simulink model "Integration_1_1"  (R2024b)
settings: Solver=VariableStepAuto  StartTime=0.0  StopTime=4  RelTol=1e-3
undefined symbols (not defined in the file): Ion, Lithium, Ts_Control
libraries: ee_lib x30, nesl_utility x24, spsSeriesRLCBranchLib x22, simulink x21, slpidlib x18, spsParallelRLCBranchLib x18, spsCurrentVoltageSimscapeInterfaceLib x18, powerlib_extras x18, spsThreePhaseVIMeasurementLib x7, spsGroundLib x7, spsThreePhaseSeriesRLCBranchLib x7, spsBoostConverterLib x6
(part 2 of 5)

== system Integration_1_1/Subsystem20 ==
  Series RLC Branch1 : spsSeriesRLCBranchLib/Series RLC Branch  LConnTagsString=__new0  RConnTagsString=__new0  BranchType=C  Resistance=10  Inductance=1e-3  SetiL0=off  InitialCurrent=0  Capacitance=1.316e-6  Setx0=off  InitialVoltage=0  Measurements=None
  Series RLC Branch2 : spsSeriesRLCBranchLib/Series RLC Branch  LConnTagsString=__new0  RConnTagsString=__new0  BranchType=C  Resistance=10  Inductance=1e-3  SetiL0=off  InitialCurrent=0  Capacitance=1.316e-6  Setx0=off  InitialVoltage=0  Measurements=None
  Series RLC Branch3 : spsSeriesRLCBranchLib/Series RLC Branch  LConnTagsString=__new0  RConnTagsString=__new0  BranchType=C  Resistance=10  Inductance=1e-3  SetiL0=off  InitialCurrent=0  Capacitance=1.316e-6  Setx0=off  InitialVoltage=0  Measurements=None
  Three-Phase Series RLC Branch1 : spsThreePhaseSeriesRLCBranchLib/Three-Phase Series RLC Branch  LConnTagsString=A|B|C  RConnTagsString=A|B|C  BranchType=L  Resistance=1  Inductance=3*2.309e-3  Capacitance=1e-6  Measurements=None
  A : PMIOPort  Side=Left
  B : PMIOPort  Port=2  Side=Left
  C : PMIOPort  Port=3  Side=Left
  a : PMIOPort  Port=4  Side=Right
  b : PMIOPort  Port=5  Side=Right
  c : PMIOPort  Port=6  Side=Right
  connections:
  Series RLC Branch2/LConn1 -- Series RLC Branch1/RConn1 -- c/RConn1 -- Three-Phase Series RLC Branch1/RConn3
  Three-Phase Series RLC Branch1/LConn3 -- C/RConn1
  Three-Phase Series RLC Branch1/LConn2 -- B/RConn1
  Three-Phase Series RLC Branch1/LConn1 -- A/RConn1
  Series RLC Branch2/RConn1 -- a/RConn1 -- Three-Phase Series RLC Branch1/RConn1 -- Series RLC Branch3/LConn1
  Series RLC Branch3/RConn1 -- b/RConn1 -- Three-Phase Series RLC Branch1/RConn2 -- Series RLC Branch1/LConn1

== system Integration_1_1/Subsystem3 ==
  Current-Voltage Simscape Interface : spsCurrentVoltageSimscapeInterfaceLib/Current-Voltage Simscape Interface  DFT=off  FMode=Low pass filter (continuous)  T=1e-4  Ts=50e-6  i0=0  v0=0  Sd=Specialized Power Systems side  Measurements=off
  Current-Voltage Simscape Interface1 : spsCurrentVoltageSimscapeInterfaceLib/Current-Voltage Simscape Interface  DFT=off  FMode=Low pass filter (continuous)  T=1e-4  Ts=50e-6  i0=0  v0=0  Sd=Specialized Power Systems side  Measurements=off
  Current-Voltage Simscape Interface2 : spsCurrentVoltageSimscapeInterfaceLib/Current-Voltage Simscape Interface  DFT=off  FMode=Low pass filter (continuous)  T=1e-4  Ts=50e-6  i0=0  v0=0  Sd=Specialized Power Systems side  Measurements=off
  Demux2 : Demux  Outputs=2
  Dynamic Load (Three-Phase) : ee_lib/Passive/Dynamic Load (Three-Phase)  port_option=ee.enum.threePhasePort.composite  FRated=50 Hz  Vline_rms_min=400 V  tau=0.01 s  Vline_rms_ini=400 V  Vang_ini=0 deg  gmin=0 S  fault_action=simscape.enum.assert.action.none  t_fault=1 s
      settings: InternalSimscapePortConfiguration="{\"Bottom\":[],\"Left\":[{\"id\":\"N\",\"label\":\"~\",\"type\":\"foundation.electrical.three_phase\"}],\"Right\":[],\"Top\":[{\"id\":\"P\",\"label\":\"P\",\"type\":\"input\"},{\"id\":\"Q\",\"label\":\"Q\",\"type\":\"input\"}]}"
  From Workspace5 : FromWorkspace  VariableName=load_data_32  SampleTime=0.01
  Ground3 : spsGroundLib/Ground  LConnTagsString=a
  Grounded Neutral (Three-Phase) : ee_lib/Connectors & References/Grounded Neutral (Three-Phase)
  PS-Simulink Converter : nesl_utility/PS-Simulink Converter  PhysicalDomain=network_engine_domain  SubClassName=ps_output  LeftPortType=input  RightPortType=output  PseudoPeriodic=off  Frequencies=[]  VectorFormat=inherit  Unit=inherit  AffineConversion=off
  Phase Splitter : ee_lib/Connectors & References/Phase Splitter
  Phase Splitter1 : ee_lib/Connectors & References/Phase Splitter
  Power Sensor (Three-Phase) : ee_lib/Sensors & Transducers/Power Sensor (Three-Phase)  load_type=ee.enum.passive.type_balanced.unbalanced  f0=50 Hz  config=ee.enum.with_neutral.no  rho=1
      settings: InternalSimscapePortConfiguration="{\"Bottom\":[],\"Left\":[{\"id\":\"N1\",\"label\":\"~1\",\"type\":\"foundation.electrical.three_phase\"}],\"Right\":[{\"id\":\"N2\",\"label\":\"~2\",\"type\":\"foundation.electrical.three_phase\"}],\"Top\":[{\"id\":\"Pm\",\"label\":\"P\",\"type\":\"output\"},{\"id\":\"Qm\",\"label\":\"Q\",\"type\":\"output\"}]}"
  Simulink-PS Converter : nesl_utility/Simulink-PS Converter  PhysicalDomain=network_engine_domain  SubClassName=ps_input  LeftPortType=input  RightPortType=output  PseudoPeriodic=off  Frequencies=[]  NoiseDistribution=none  NoiseParameters=[]  Unit=1  AffineConversion=off  FilteringAndDerivatives=provide  SimscapeFilterOrder=1  InputFilterTimeConstant=0.001  UdotUserProvided=0
  Simulink-PS Converter1 : nesl_utility/Simulink-PS Converter  PhysicalDomain=network_engine_domain  SubClassName=ps_input  LeftPortType=input  RightPortType=output  PseudoPeriodic=off  Frequencies=[]  NoiseDistribution=none  NoiseParameters=[]  Unit=1  AffineConversion=off  FilteringAndDerivatives=provide  SimscapeFilterOrder=1  InputFilterTimeConstant=0.001  UdotUserProvided=0
  Solver Configuration : nesl_utility/Solver Configuration  PhysicalDomain=network_engine_domain  SubClassName=solver  LeftPortType=input  RightPortType=generic  Tones=[]  Harmonics=[]  SimulateNoise=off  Profile=off  UseLocalSampling=off  EnableSwitchedLinearOptims=on  FrequencyDomain=off  UseCCode=off  RelTol=0.001  AbsTol=0.001  MinStep=1e-09  ToWorkspace=off  RevertToSquareIcSolve=off  NumHomotopyIterations=100  PhasorMode=off  PhasorModeNumHarmonics=1  ConsistencySolver=NEWTON_XTOL_AFTER_FTOL  IndexReductionMethod=DerivativeReplacement  DoDC=on  ResidualTolerance=1e-09  ConsistencyTolSource=GLOBAL  ConsistencyAbsTol=0.001  ConsistencyRelTol=0.001  ConsistencyTolFactor=0.001  UseLocalSolver=off  LocalSolverChoice=NE_BACKWARD_EULER_ADVANCER  ResolveIndetEquations=on  FunctionEvalNumThread=1  LocalSolverSampleTime=0.0001  DoFixedCost=off  MaxNonlinIter=3  MaxModeIter=2  ComputeImpulses=off  ImpulseIterations=2  LinearAlgebra=Sparse  LinearAlgebraNumThread=0  EquationFormulation=NE_TIME_EF  DelaysMemoryBudget=1024  AutomaticFiltering=off  FilteringTimeConstant=0.001  PartitionStorageMethod=AS_NEEDED  PartitionMemoryBudget=1024  PartitionMethod=ROBUST  MultibodyUseLocalSolver=off  MultibodyLocalSolverChoice=ODE1  MultibodyLocalSolverSampleTime=0.001
  A1 : PMIOPort  Side=Left
  B1 : PMIOPort  Port=2  Side=Left
  C1 : PMIOPort  Port=3  Side=Left
  tag scope: load_4_P=global
  wires:
  Demux2/1 -> Simulink-PS Converter/1
  PS-Simulink Converter/1 -> [load_4_P]
  Demux2/2 -> Simulink-PS Converter1/1
  From Workspace5/1 -> Demux2/1
  connections:
  C1/RConn1 -- Current-Voltage Simscape Interface2/LConn1
  Current-Voltage Simscape Interface/LConn2 -- Ground3/LConn1 -- Current-Voltage Simscape Interface2/LConn2 -- Current-Voltage Simscape Interface1/LConn2
  Current-Voltage Simscape Interface1/LConn1 -- B1/RConn1
  A1/RConn1 -- Current-Voltage Simscape Interface/LConn1
  Dynamic Load (Three-Phase)/LConn2 -- Simulink-PS Converter/RConn1
  PS-Simulink Converter/LConn1 -- Power Sensor (Three-Phase)/LConn2
  Current-Voltage Simscape Interface/RConn2 -- Phase Splitter1/RConn1
  Grounded Neutral (Three-Phase)/LConn1 -- Phase Splitter1/LConn1
  Dynamic Load (Three-Phase)/LConn3 -- Simulink-PS Converter1/RConn1
  Current-Voltage Simscape Interface/RConn1 -- Phase Splitter/RConn1
  Current-Voltage Simscape Interface2/RConn1 -- Phase Splitter/RConn3
  Current-Voltage Simscape Interface1/RConn1 -- Phase Splitter/RConn2
  Dynamic Load (Three-Phase)/LConn1 -- Power Sensor (Three-Phase)/RConn1
  Current-Voltage Simscape Interface2/RConn2 -- Phase Splitter1/RConn3
  Current-Voltage Simscape Interface1/RConn2 -- Phase Splitter1/RConn2
  Phase Splitter/LConn1 -- Solver Configuration/RConn1 -- Power Sensor (Three-Phase)/LConn1

== system Integration_1_1/Subsystem4 ==
  Current-Voltage Simscape Interface : spsCurrentVoltageSimscapeInterfaceLib/Current-Voltage Simscape Interface  DFT=off  FMode=Low pass filter (continuous)  T=1e-4  Ts=50e-6  i0=0  v0=0  Sd=Specialized Power Systems side  Measurements=off
  Current-Voltage Simscape Interface1 : spsCurrentVoltageSimscapeInterfaceLib/Current-Voltage Simscape Interface  DFT=off  FMode=Low pass filter (continuous)  T=1e-4  Ts=50e-6  i0=0  v0=0  Sd=Specialized Power Systems side  Measurements=off
  Current-Voltage Simscape Interface2 : spsCurrentVoltageSimscapeInterfaceLib/Current-Voltage Simscape Interface  DFT=off  FMode=Low pass filter (continuous)  T=1e-4  Ts=50e-6  i0=0  v0=0  Sd=Specialized Power Systems side  Measurements=off
  Demux2 : Demux  Outputs=2
  Dynamic Load (Three-Phase) : ee_lib/Passive/Dynamic Load (Three-Phase)  port_option=ee.enum.threePhasePort.composite  FRated=50 Hz  Vline_rms_min=400 V  tau=0.01 s  Vline_rms_ini=400 V  Vang_ini=0 deg  gmin=0 S  fault_action=simscape.enum.assert.action.none  t_fault=1 s
      settings: InternalSimscapePortConfiguration="{\"Bottom\":[],\"Left\":[{\"id\":\"N\",\"label\":\"~\",\"type\":\"foundation.electrical.three_phase\"}],\"Right\":[],\"Top\":[{\"id\":\"P\",\"label\":\"P\",\"type\":\"input\"},{\"id\":\"Q\",\"label\":\"Q\",\"type\":\"input\"}]}"
  From Workspace5 : FromWorkspace  VariableName=load_data_27  SampleTime=0.01
  Ground3 : spsGroundLib/Ground  LConnTagsString=a
  Grounded Neutral (Three-Phase) : ee_lib/Connectors & References/Grounded Neutral (Three-Phase)
  PS-Simulink Converter : nesl_utility/PS-Simulink Converter  PhysicalDomain=network_engine_domain  SubClassName=ps_output  LeftPortType=input  RightPortType=output  PseudoPeriodic=off  Frequencies=[]  VectorFormat=inherit  Unit=inherit  AffineConversion=off
  Phase Splitter : ee_lib/Connectors & References/Phase Splitter
  Phase Splitter1 : ee_lib/Connectors & References/Phase Splitter
  Power Sensor (Three-Phase) : ee_lib/Sensors & Transducers/Power Sensor (Three-Phase)  load_type=ee.enum.passive.type_balanced.unbalanced  f0=50 Hz  config=ee.enum.with_neutral.no  rho=1
      settings: InternalSimscapePortConfiguration="{\"Bottom\":[],\"Left\":[{\"id\":\"N1\",\"label\":\"~1\",\"type\":\"foundation.electrical.three_phase\"}],\"Right\":[{\"id\":\"N2\",\"label\":\"~2\",\"type\":\"foundation.electrical.three_phase\"}],\"Top\":[{\"id\":\"Pm\",\"label\":\"P\",\"type\":\"output\"},{\"id\":\"Qm\",\"label\":\"Q\",\"type\":\"output\"}]}"
  Simulink-PS Converter : nesl_utility/Simulink-PS Converter  PhysicalDomain=network_engine_domain  SubClassName=ps_input  LeftPortType=input  RightPortType=output  PseudoPeriodic=off  Frequencies=[]  NoiseDistribution=none  NoiseParameters=[]  Unit=1  AffineConversion=off  FilteringAndDerivatives=provide  SimscapeFilterOrder=1  InputFilterTimeConstant=0.001  UdotUserProvided=0
  Simulink-PS Converter1 : nesl_utility/Simulink-PS Converter  PhysicalDomain=network_engine_domain  SubClassName=ps_input  LeftPortType=input  RightPortType=output  PseudoPeriodic=off  Frequencies=[]  NoiseDistribution=none  NoiseParameters=[]  Unit=1  AffineConversion=off  FilteringAndDerivatives=provide  SimscapeFilterOrder=1  InputFilterTimeConstant=0.001  UdotUserProvided=0
  Solver Configuration : nesl_utility/Solver Configuration  PhysicalDomain=network_engine_domain  SubClassName=solver  LeftPortType=input  RightPortType=generic  Tones=[]  Harmonics=[]  SimulateNoise=off  Profile=off  UseLocalSampling=off  EnableSwitchedLinearOptims=on  FrequencyDomain=off  UseCCode=off  RelTol=0.001  AbsTol=0.001  MinStep=1e-09  ToWorkspace=off  RevertToSquareIcSolve=off  NumHomotopyIterations=100  PhasorMode=off  PhasorModeNumHarmonics=1  ConsistencySolver=NEWTON_XTOL_AFTER_FTOL  IndexReductionMethod=DerivativeReplacement  DoDC=on  ResidualTolerance=1e-09  ConsistencyTolSource=GLOBAL  ConsistencyAbsTol=0.001  ConsistencyRelTol=0.001  ConsistencyTolFactor=0.001  UseLocalSolver=off  LocalSolverChoice=NE_BACKWARD_EULER_ADVANCER  ResolveIndetEquations=on  FunctionEvalNumThread=1  LocalSolverSampleTime=0.0001  DoFixedCost=off  MaxNonlinIter=3  MaxModeIter=2  ComputeImpulses=off  ImpulseIterations=2  LinearAlgebra=Sparse  LinearAlgebraNumThread=0  EquationFormulation=NE_TIME_EF  DelaysMemoryBudget=1024  AutomaticFiltering=off  FilteringTimeConstant=0.001  PartitionStorageMethod=AS_NEEDED  PartitionMemoryBudget=1024  PartitionMethod=ROBUST  MultibodyUseLocalSolver=off  MultibodyLocalSolverChoice=ODE1  MultibodyLocalSolverSampleTime=0.001
  A1 : PMIOPort  Side=Left
  B1 : PMIOPort  Port=2  Side=Left
  C1 : PMIOPort  Port=3  Side=Left
  tag scope: load_2_P=global
  wires:
  Demux2/1 -> Simulink-PS Converter/1
  PS-Simulink Converter/1 -> [load_2_P]
  Demux2/2 -> Simulink-PS Converter1/1
  From Workspace5/1 -> Demux2/1
  connections:
  C1/RConn1 -- Current-Voltage Simscape Interface2/LConn1
  Current-Voltage Simscape Interface/LConn2 -- Ground3/LConn1 -- Current-Voltage Simscape Interface2/LConn2 -- Current-Voltage Simscape Interface1/LConn2
  Current-Voltage Simscape Interface1/LConn1 -- B1/RConn1
  A1/RConn1 -- Current-Voltage Simscape Interface/LConn1
  Dynamic Load (Three-Phase)/LConn2 -- Simulink-PS Converter/RConn1
  PS-Simulink Converter/LConn1 -- Power Sensor (Three-Phase)/LConn2
  Current-Voltage Simscape Interface/RConn2 -- Phase Splitter1/RConn1
  Grounded Neutral (Three-Phase)/LConn1 -- Phase Splitter1/LConn1
  Dynamic Load (Three-Phase)/LConn3 -- Simulink-PS Converter1/RConn1
  Current-Voltage Simscape Interface/RConn1 -- Phase Splitter/RConn1
  Current-Voltage Simscape Interface2/RConn1 -- Phase Splitter/RConn3
  Current-Voltage Simscape Interface1/RConn1 -- Phase Splitter/RConn2
  Dynamic Load (Three-Phase)/LConn1 -- Power Sensor (Three-Phase)/RConn1
  Current-Voltage Simscape Interface2/RConn2 -- Phase Splitter1/RConn3
  Current-Voltage Simscape Interface1/RConn2 -- Phase Splitter1/RConn2
  Phase Splitter/LConn1 -- Solver Configuration/RConn1 -- Power Sensor (Three-Phase)/LConn1

== system Integration_1_1/Subsystem5 ==
  B2 : spsThreePhaseVIMeasurementLib/Three-Phase V-I Measurement  VoltageMeasurement=phase-to-ground  SetLabelV=on  LabelV=Vabc_B2  Vpu=off  VpuLL=off  CurrentMeasurement=yes  SetLabelI=on  LabelI=Iabc_B2  Ipu=off  Pbase=100e6  Vbase=500e3  OutputType=Magnitude  PhasorSimulation=off  PSBequivalent=0
  Ground : spsGroundLib/Ground  LConnTagsString=a
  "Grounding Transformer " : spsGroundingTransformerLib/Grounding Transformer   UNITS=SI  NominalPower="[3e3   50]"  NominalVoltage=0.4e3  ZeroSequenceImpedance_pu=[0.025 0.75]  MagnetizationBranch_pu=[500 500]  ZeroSequenceImpedance_SI=[1.3333 40]  MagnetizationBranch_SI=[26667 26667]  Measurements=All voltages and currents
      settings: LibrarySourceBlock=|
      | sps_lib/Power Grid Elements/Grounding
      | Transformer
  Three-Phase Series RLC Branch3 : spsThreePhaseSeriesRLCBranchLib/Three-Phase Series RLC Branch  LConnTagsString=A|B|C  RConnTagsString=A|B|C  BranchType=RL  Resistance=0.02  Inductance=1e-3  Capacitance=1e-6  Measurements=None
  Three-Phase Series RLC Load : spsThreePhaseSeriesRLCLoadLib/Three-Phase Series RLC Load  LConnTagsString=A|B|C  Configuration=Y (grounded)  NominalVoltage=400  Vabc=[1e3 1e3 1e3]  Vabcp=[1e3 1e3 1e3]  NominalFrequency=50  UnbalancedPower=off  ActivePower=0  InductivePower=0  CapacitivePower=1e3  Pabc=[10e3 9e3 11e3]  QLabc=[100 90 110]  QCabc=[100 90 110]  Pabcp=[10e3 9e3 11e3]  QLabcp=[100 90 110]  QCabcp=[100 90 110]  Measurements=None  LoadType=constant Z
  Three-Phase Series RLC Load1 : spsThreePhaseSeriesRLCLoadLib/Three-Phase Series RLC Load  LConnTagsString=A|B|C  Configuration=Y (grounded)  NominalVoltage=400  Vabc=[1e3 1e3 1e3]  Vabcp=[1e3 1e3 1e3]  NominalFrequency=50  UnbalancedPower=off  ActivePower=10  InductivePower=0  CapacitivePower=0  Pabc=[10e3 9e3 11e3]  QLabc=[100 90 110]  QCabc=[100 90 110]  Pabcp=[10e3 9e3 11e3]  QLabcp=[100 90 110]  QCabcp=[100 90 110]  Measurements=None  LoadType=constant Z
  Three-Phase Source : spsThreePhaseSourceLib/Three-Phase Source  InternalConnection=Yg  VoltagePhases=off  Voltage=400  PhaseAngle=0  Voltage_phases=[25e3 25e3 25e3]/sqrt(3)  PhaseAngles_phases=[0 -120 +120]  Frequency=50  NonIdealSource=on  SpecifyImpedance=on  Resistance=0.0113  Inductance=36e-6  ShortCircuitLevel=10e6  BaseVoltage=400  XRratio=6  BusType=swing  Pref=10e3  Qref=0  Prefabc=[10e3, 10e3, 10e3]  Qrefabc=[0, 0, 0]  Qmin=-inf  Qmax=inf
  A : PMIOPort  Side=Left
  B : PMIOPort  Port=2  Side=Left
  C : PMIOPort  Port=3  Side=Left
  connections:
  "Grounding Transformer "/RConn1 -- Ground/LConn1
  Three-Phase Series RLC Load/LConn1 -- Three-Phase Series RLC Branch3/RConn1 -- Three-Phase Source/RConn1
  Three-Phase Series RLC Load/LConn2 -- Three-Phase Series RLC Branch3/RConn2 -- Three-Phase Source/RConn2
  Three-Phase Series RLC Load/LConn3 -- Three-Phase Series RLC Branch3/RConn3 -- Three-Phase Source/RConn3
  "Grounding Transformer "/LConn1 -- B2/LConn1 -- Three-Phase Series RLC Load1/LConn1 -- Three-Phase Series RLC Branch3/LConn1
  "Grounding Transformer "/LConn2 -- Three-Phase Series RLC Load1/LConn2 -- B2/LConn2 -- Three-Phase Series RLC Branch3/LConn2
  "Grounding Transformer "/LConn3 -- Three-Phase Series RLC Load1/LConn3 -- B2/LConn3 -- Three-Phase Series RLC Branch3/LConn3
  B2/RConn3 -- C/RConn1
  B2/RConn2 -- B/RConn1
  B2/RConn1 -- A/RConn1

== system Integration_1_1/Subsystem6 ==
  Current-Voltage Simscape Interface : spsCurrentVoltageSimscapeInterfaceLib/Current-Voltage Simscape Interface  DFT=off  FMode=Low pass filter (continuous)  T=1e-4  Ts=50e-6  i0=0  v0=0  Sd=Specialized Power Systems side  Measurements=off
  Current-Voltage Simscape Interface1 : spsCurrentVoltageSimscapeInterfaceLib/Current-Voltage Simscape Interface  DFT=off  FMode=Low pass filter (continuous)  T=1e-4  Ts=50e-6  i0=0  v0=0  Sd=Specialized Power Systems side  Measurements=off
  Current-Voltage Simscape Interface2 : spsCurrentVoltageSimscapeInterfaceLib/Current-Voltage Simscape Interface  DFT=off  FMode=Low pass filter (continuous)  T=1e-4  Ts=50e-6  i0=0  v0=0  Sd=Specialized Power Systems side  Measurements=off
  Demux2 : Demux  Outputs=2
  Dynamic Load (Three-Phase) : ee_lib/Passive/Dynamic Load (Three-Phase)  port_option=ee.enum.threePhasePort.composite  FRated=50 Hz  Vline_rms_min=400 V  tau=0.01 s  Vline_rms_ini=400 V  Vang_ini=0 deg  gmin=0 S  fault_action=simscape.enum.assert.action.none  t_fault=1 s
      settings: InternalSimscapePortConfiguration="{\"Bottom\":[],\"Left\":[{\"id\":\"N\",\"label\":\"~\",\"type\":\"foundation.electrical.three_phase\"}],\"Right\":[],\"Top\":[{\"id\":\"P\",\"label\":\"P\",\"type\":\"input\"},{\"id\":\"Q\",\"label\":\"Q\",\"type\":\"input\"}]}"
  From Workspace5 : FromWorkspace  VariableName=load_data_30  SampleTime=0.01
  Ground3 : spsGroundLib/Ground  LConnTagsString=a
  Grounded Neutral (Three-Phase) : ee_lib/Connectors & References/Grounded Neutral (Three-Phase)
  PS-Simulink Converter : nesl_utility/PS-Simulink Converter  PhysicalDomain=network_engine_domain  SubClassName=ps_output  LeftPortType=input  RightPortType=output  PseudoPeriodic=off  Frequencies=[]  VectorFormat=inherit  Unit=inherit  AffineConversion=off
  Phase Splitter : ee_lib/Connectors & References/Phase Splitter
  Phase Splitter1 : ee_lib/Connectors & References/Phase Splitter
  Power Sensor (Three-Phase) : ee_lib/Sensors & Transducers/Power Sensor (Three-Phase)  load_type=ee.enum.passive.type_balanced.unbalanced  f0=50 Hz  config=ee.enum.with_neutral.no  rho=1
      settings: InternalSimscapePortConfiguration="{\"Bottom\":[],\"Left\":[{\"id\":\"N1\",\"label\":\"~1\",\"type\":\"foundation.electrical.three_phase\"}],\"Right\":[{\"id\":\"N2\",\"label\":\"~2\",\"type\":\"foundation.electrical.three_phase\"}],\"Top\":[{\"id\":\"Pm\",\"label\":\"P\",\"type\":\"output\"},{\"id\":\"Qm\",\"label\":\"Q\",\"type\":\"output\"}]}"
  Simulink-PS Converter : nesl_utility/Simulink-PS Converter  PhysicalDomain=network_engine_domain  SubClassName=ps_input  LeftPortType=input  RightPortType=output  PseudoPeriodic=off  Frequencies=[]  NoiseDistribution=none  NoiseParameters=[]  Unit=1  AffineConversion=off  FilteringAndDerivatives=provide  SimscapeFilterOrder=1  InputFilterTimeConstant=0.001  UdotUserProvided=0
  Simulink-PS Converter1 : nesl_utility/Simulink-PS Converter  PhysicalDomain=network_engine_domain  SubClassName=ps_input  LeftPortType=input  RightPortType=output  PseudoPeriodic=off  Frequencies=[]  NoiseDistribution=none  NoiseParameters=[]  Unit=1  AffineConversion=off  FilteringAndDerivatives=provide  SimscapeFilterOrder=1  InputFilterTimeConstant=0.001  UdotUserProvided=0
  Solver Configuration : nesl_utility/Solver Configuration  PhysicalDomain=network_engine_domain  SubClassName=solver  LeftPortType=input  RightPortType=generic  Tones=[]  Harmonics=[]  SimulateNoise=off  Profile=off  UseLocalSampling=off  EnableSwitchedLinearOptims=on  FrequencyDomain=off  UseCCode=off  RelTol=0.001  AbsTol=0.001  MinStep=1e-09  ToWorkspace=off  RevertToSquareIcSolve=off  NumHomotopyIterations=100  PhasorMode=off  PhasorModeNumHarmonics=1  ConsistencySolver=NEWTON_XTOL_AFTER_FTOL  IndexReductionMethod=DerivativeReplacement  DoDC=on  ResidualTolerance=1e-09  ConsistencyTolSource=GLOBAL  ConsistencyAbsTol=0.001  ConsistencyRelTol=0.001  ConsistencyTolFactor=0.001  UseLocalSolver=off  LocalSolverChoice=NE_BACKWARD_EULER_ADVANCER  ResolveIndetEquations=on  FunctionEvalNumThread=1  LocalSolverSampleTime=0.0001  DoFixedCost=off  MaxNonlinIter=3  MaxModeIter=2  ComputeImpulses=off  ImpulseIterations=2  LinearAlgebra=Sparse  LinearAlgebraNumThread=0  EquationFormulation=NE_TIME_EF  DelaysMemoryBudget=1024  AutomaticFiltering=off  FilteringTimeConstant=0.001  PartitionStorageMethod=AS_NEEDED  PartitionMemoryBudget=1024  PartitionMethod=ROBUST  MultibodyUseLocalSolver=off  MultibodyLocalSolverChoice=ODE1  MultibodyLocalSolverSampleTime=0.001
  A1 : PMIOPort  Side=Left
  B1 : PMIOPort  Port=2  Side=Left
  C1 : PMIOPort  Port=3  Side=Left
  tag scope: load_3_P=global
  wires:
  From Workspace5/1 -> Demux2/1
  Demux2/2 -> Simulink-PS Converter1/1
  PS-Simulink Converter/1 -> [load_3_P]
  Demux2/1 -> Simulink-PS Converter/1
  connections:
  Power Sensor (Three-Phase)/LConn1 -- Solver Configuration/RConn1 -- Phase Splitter/LConn1
  Current-Voltage Simscape Interface1/RConn2 -- Phase Splitter1/RConn2
  Current-Voltage Simscape Interface2/RConn2 -- Phase Splitter1/RConn3
  Dynamic Load (Three-Phase)/LConn1 -- Power Sensor (Three-Phase)/RConn1
  Current-Voltage Simscape Interface1/RConn1 -- Phase Splitter/RConn2
  Current-Voltage Simscape Interface2/RConn1 -- Phase Splitter/RConn3
  Current-Voltage Simscape Interface/RConn1 -- Phase Splitter/RConn1
  Dynamic Load (Three-Phase)/LConn3 -- Simulink-PS Converter1/RConn1
  Grounded Neutral (Three-Phase)/LConn1 -- Phase Splitter1/LConn1
  Current-Voltage Simscape Interface/RConn2 -- Phase Splitter1/RConn1
  PS-Simulink Converter/LConn1 -- Power Sensor (Three-Phase)/LConn2
  Dynamic Load (Three-Phase)/LConn2 -- Simulink-PS Converter/RConn1
  A1/RConn1 -- Current-Voltage Simscape Interface/LConn1
  Current-Voltage Simscape Interface1/LConn1 -- B1/RConn1
  Current-Voltage Simscape Interface1/LConn2 -- Current-Voltage Simscape Interface2/LConn2 -- Ground3/LConn1 -- Current-Voltage Simscape Interface/LConn2
  C1/RConn1 -- Current-Voltage Simscape Interface2/LConn1

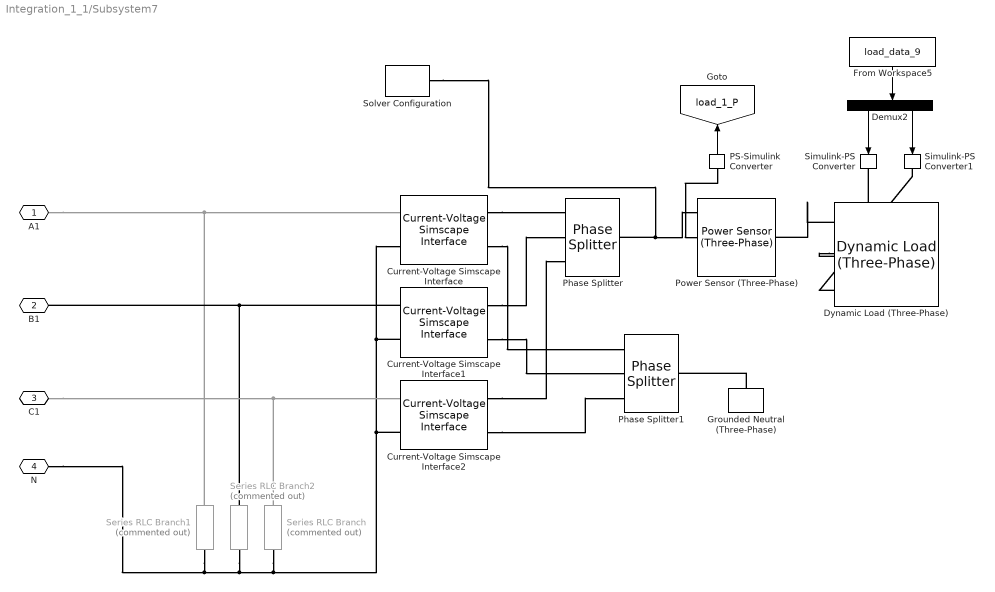
== system Integration_1_1/Subsystem7 ==
  Current-Voltage Simscape Interface : spsCurrentVoltageSimscapeInterfaceLib/Current-Voltage Simscape Interface  DFT=off  FMode=Low pass filter (continuous)  T=1e-4  Ts=50e-6  i0=0  v0=0  Sd=Specialized Power Systems side  Measurements=off
  Current-Voltage Simscape Interface1 : spsCurrentVoltageSimscapeInterfaceLib/Current-Voltage Simscape Interface  DFT=off  FMode=Low pass filter (continuous)  T=1e-4  Ts=50e-6  i0=0  v0=0  Sd=Specialized Power Systems side  Measurements=off
  Current-Voltage Simscape Interface2 : spsCurrentVoltageSimscapeInterfaceLib/Current-Voltage Simscape Interface  DFT=off  FMode=Low pass filter (continuous)  T=1e-4  Ts=50e-6  i0=0  v0=0  Sd=Specialized Power Systems side  Measurements=off
  Demux2 : Demux  Outputs=2
  Dynamic Load (Three-Phase) : ee_lib/Passive/Dynamic Load (Three-Phase)  port_option=ee.enum.threePhasePort.composite  FRated=50 Hz  Vline_rms_min=400 V  tau=0.01 s  Vline_rms_ini=400 V  Vang_ini=0 deg  gmin=0 S  fault_action=simscape.enum.assert.action.none  t_fault=1 s
      settings: InternalSimscapePortConfiguration="{\"Bottom\":[],\"Left\":[{\"id\":\"N\",\"label\":\"~\",\"type\":\"foundation.electrical.three_phase\"}],\"Right\":[],\"Top\":[{\"id\":\"P\",\"label\":\"P\",\"type\":\"input\"},{\"id\":\"Q\",\"label\":\"Q\",\"type\":\"input\"}]}"
  From Workspace5 : FromWorkspace  VariableName=load_data_9  SampleTime=0.01
  Grounded Neutral (Three-Phase) : ee_lib/Connectors & References/Grounded Neutral (Three-Phase)
  PS-Simulink Converter : nesl_utility/PS-Simulink Converter  PhysicalDomain=network_engine_domain  SubClassName=ps_output  LeftPortType=input  RightPortType=output  PseudoPeriodic=off  Frequencies=[]  VectorFormat=inherit  Unit=inherit  AffineConversion=off
  Phase Splitter : ee_lib/Connectors & References/Phase Splitter
  Phase Splitter1 : ee_lib/Connectors & References/Phase Splitter
  Power Sensor (Three-Phase) : ee_lib/Sensors & Transducers/Power Sensor (Three-Phase)  load_type=ee.enum.passive.type_balanced.unbalanced  f0=50 Hz  config=ee.enum.with_neutral.no  rho=1
      settings: InternalSimscapePortConfiguration="{\"Bottom\":[],\"Left\":[{\"id\":\"N1\",\"label\":\"~1\",\"type\":\"foundation.electrical.three_phase\"}],\"Right\":[{\"id\":\"N2\",\"label\":\"~2\",\"type\":\"foundation.electrical.three_phase\"}],\"Top\":[{\"id\":\"Pm\",\"label\":\"P\",\"type\":\"output\"},{\"id\":\"Qm\",\"label\":\"Q\",\"type\":\"output\"}]}"
  Series RLC Branch : spsSeriesRLCBranchLib/Series RLC Branch  Commented=on  LConnTagsString=__new0  RConnTagsString=__new0  BranchType=R  Resistance=1  Inductance=1e-3  SetiL0=off  InitialCurrent=0  Capacitance=1e-6  Setx0=off  InitialVoltage=0  Measurements=None
  Series RLC Branch1 : spsSeriesRLCBranchLib/Series RLC Branch  Commented=on  LConnTagsString=__new0  RConnTagsString=__new0  BranchType=R  Resistance=1  Inductance=1e-3  SetiL0=off  InitialCurrent=0  Capacitance=1e-6  Setx0=off  InitialVoltage=0  Measurements=None
  Series RLC Branch2 : spsSeriesRLCBranchLib/Series RLC Branch  Commented=on  LConnTagsString=__new0  RConnTagsString=__new0  BranchType=R  Resistance=1  Inductance=1e-3  SetiL0=off  InitialCurrent=0  Capacitance=1e-6  Setx0=off  InitialVoltage=0  Measurements=None
  Simulink-PS Converter : nesl_utility/Simulink-PS Converter  PhysicalDomain=network_engine_domain  SubClassName=ps_input  LeftPortType=input  RightPortType=output  PseudoPeriodic=off  Frequencies=[]  NoiseDistribution=none  NoiseParameters=[]  Unit=1  AffineConversion=off  FilteringAndDerivatives=provide  SimscapeFilterOrder=1  InputFilterTimeConstant=0.001  UdotUserProvided=0
  Simulink-PS Converter1 : nesl_utility/Simulink-PS Converter  PhysicalDomain=network_engine_domain  SubClassName=ps_input  LeftPortType=input  RightPortType=output  PseudoPeriodic=off  Frequencies=[]  NoiseDistribution=none  NoiseParameters=[]  Unit=1  AffineConversion=off  FilteringAndDerivatives=provide  SimscapeFilterOrder=1  InputFilterTimeConstant=0.001  UdotUserProvided=0
  Solver Configuration : nesl_utility/Solver Configuration  PhysicalDomain=network_engine_domain  SubClassName=solver  LeftPortType=input  RightPortType=generic  Tones=[]  Harmonics=[]  SimulateNoise=off  Profile=off  UseLocalSampling=off  EnableSwitchedLinearOptims=on  FrequencyDomain=off  UseCCode=off  RelTol=0.001  AbsTol=0.001  MinStep=1e-09  ToWorkspace=off  RevertToSquareIcSolve=off  NumHomotopyIterations=100  PhasorMode=off  PhasorModeNumHarmonics=1  ConsistencySolver=NEWTON_XTOL_AFTER_FTOL  IndexReductionMethod=DerivativeReplacement  DoDC=on  ResidualTolerance=1e-09  ConsistencyTolSource=GLOBAL  ConsistencyAbsTol=0.001  ConsistencyRelTol=0.001  ConsistencyTolFactor=0.001  UseLocalSolver=off  LocalSolverChoice=NE_BACKWARD_EULER_ADVANCER  ResolveIndetEquations=on  FunctionEvalNumThread=1  LocalSolverSampleTime=0.0001  DoFixedCost=off  MaxNonlinIter=3  MaxModeIter=2  ComputeImpulses=off  ImpulseIterations=2  LinearAlgebra=Sparse  LinearAlgebraNumThread=0  EquationFormulation=NE_TIME_EF  DelaysMemoryBudget=1024  AutomaticFiltering=off  FilteringTimeConstant=0.001  PartitionStorageMethod=AS_NEEDED  PartitionMemoryBudget=1024  PartitionMethod=ROBUST  MultibodyUseLocalSolver=off  MultibodyLocalSolverChoice=ODE1  MultibodyLocalSolverSampleTime=0.001
  A1 : PMIOPort  Side=Left
  B1 : PMIOPort  Port=2  Side=Left
  C1 : PMIOPort  Port=3  Side=Left
  N : PMIOPort  Port=4  Side=Left
  tag scope: load_1_P=global
  wires:
  From Workspace5/1 -> Demux2/1
  Demux2/2 -> Simulink-PS Converter1/1
  PS-Simulink Converter/1 -> [load_1_P]
  Demux2/1 -> Simulink-PS Converter/1
  connections:
  Power Sensor (Three-Phase)/LConn1 -- Solver Configuration/RConn1 -- Phase Splitter/LConn1
  Current-Voltage Simscape Interface1/RConn2 -- Phase Splitter1/RConn2
  Current-Voltage Simscape Interface2/RConn2 -- Phase Splitter1/RConn3
  Dynamic Load (Three-Phase)/LConn1 -- Power Sensor (Three-Phase)/RConn1
  Current-Voltage Simscape Interface1/RConn1 -- Phase Splitter/RConn2
  Current-Voltage Simscape Interface2/RConn1 -- Phase Splitter/RConn3
  Current-Voltage Simscape Interface/RConn1 -- Phase Splitter/RConn1
  Dynamic Load (Three-Phase)/LConn3 -- Simulink-PS Converter1/RConn1
  Grounded Neutral (Three-Phase)/LConn1 -- Phase Splitter1/LConn1
  Current-Voltage Simscape Interface/RConn2 -- Phase Splitter1/RConn1
  PS-Simulink Converter/LConn1 -- Power Sensor (Three-Phase)/LConn2
  Dynamic Load (Three-Phase)/LConn2 -- Simulink-PS Converter/RConn1
  Series RLC Branch1/LConn1 -- Current-Voltage Simscape Interface/LConn1 -- A1/RConn1
  Current-Voltage Simscape Interface1/LConn1 -- Series RLC Branch2/LConn1 -- B1/RConn1
  Current-Voltage Simscape Interface1/LConn2 -- Series RLC Branch/RConn1 -- N/RConn1 -- Series RLC Branch1/RConn1 -- Series RLC Branch2/RConn1 -- Current-Voltage Simscape Interface2/LConn2 -- Current-Voltage Simscape Interface/LConn2
  Series RLC Branch/LConn1 -- C1/RConn1 -- Current-Voltage Simscape Interface2/LConn1

== system Integration_1_1/Subsystem8 ==
  Parallel RLC Branch : spsParallelRLCBranchLib/Parallel RLC Branch  LConnTagsString=a  RConnTagsString=__new0  BranchType=RC  Resistance=80  Inductance=1e-3  SetiL0=off  InitialCurrent=0  Capacitance=0.68e-6  Setx0=off  InitialVoltage=0  Measurements=None
  Parallel RLC Branch1 : spsParallelRLCBranchLib/Parallel RLC Branch  LConnTagsString=a  RConnTagsString=__new0  BranchType=RC  Resistance=80  Inductance=1e-3  SetiL0=off  InitialCurrent=0  Capacitance=0.68e-6  Setx0=off  InitialVoltage=0  Measurements=None
  Parallel RLC Branch2 : spsParallelRLCBranchLib/Parallel RLC Branch  LConnTagsString=a  RConnTagsString=__new0  BranchType=RC  Resistance=80  Inductance=1e-3  SetiL0=off  InitialCurrent=0  Capacitance=0.68e-6  Setx0=off  InitialVoltage=0  Measurements=None
  Three-Phase Series RLC Branch1 : spsThreePhaseSeriesRLCBranchLib/Three-Phase Series RLC Branch  LConnTagsString=A|B|C  RConnTagsString=A|B|C  BranchType=L  Resistance=1  Inductance=3*4.45e-3  Capacitance=1e-6  Measurements=None
  A : PMIOPort  Side=Left
  B : PMIOPort  Port=2  Side=Left
  C : PMIOPort  Port=3  Side=Left
  a : PMIOPort  Port=4  Side=Right
  b : PMIOPort  Port=5  Side=Right
  c : PMIOPort  Port=6  Side=Right
  connections:
  c/RConn1 -- Parallel RLC Branch2/RConn1 -- Parallel RLC Branch1/LConn1 -- Three-Phase Series RLC Branch1/RConn3
  Three-Phase Series RLC Branch1/LConn3 -- C/RConn1
  Three-Phase Series RLC Branch1/LConn2 -- B/RConn1
  Three-Phase Series RLC Branch1/LConn1 -- A/RConn1
  a/RConn1 -- Three-Phase Series RLC Branch1/RConn1 -- Parallel RLC Branch1/RConn1 -- Parallel RLC Branch/LConn1
  b/RConn1 -- Parallel RLC Branch2/LConn1 -- Parallel RLC Branch/RConn1 -- Three-Phase Series RLC Branch1/RConn2

== system Integration_1_1/Subsystem9 ==
  "  " : Inport
  Boost Converter : spsBoostConverterLib/Boost Converter  ModelType=Average model (D-controlled)  Ron=1e-3  Rs=1e6  Cs=inf  Vforward=[0,0]  Ron_Diode=1e-3  Rs_Diode=1e6  Cs_Diode=inf  Vf_Diode=1e-3  Rs_CurrentSource=inf  Ron_ACsource=1e-3
      settings: LibrarySourceBlock=sps_lib/Power Electronics/Boost Converter
  Bus Selector1 : BusSelector  OutputSignals=V_PV,I_PV
  C_in : spsSeriesRLCBranchLib/Series RLC Branch  LConnTagsString=__new0  RConnTagsString=__new0  BranchType=C  Resistance=1e-5  Inductance=1e-3  SetiL0=off  InitialCurrent=0  Capacitance=314e-6  Setx0=off  InitialVoltage=426.5  Measurements=Branch voltage and current
  Constant4 : Constant  Value=25
  Inverter ON/OFF Logic : Subsystem
  L_boost : spsSeriesRLCBranchLib/Series RLC Branch  LConnTagsString=__new0  RConnTagsString=__new0  BranchType=L  Resistance=1e-3  Inductance=157e-3  SetiL0=off  InitialCurrent=0  Capacitance=100e-6  Setx0=off  InitialVoltage=230  Measurements=None
  MPPT3 : Subsystem
  PV Array1 : spsPVArrayLib/PV Array  Npar=3  Nser=5  PlotType=array @ 1000 W/m2 & specified temperatures  S_vec="[ 1000  500  100 ]"  Temp_C_vec="[ 45 25  ]"  ModuleName=SunPower SPR-415E-WHT-D  PlotWhenSelected=off  Pm=414.801  Ncell=128  Voc=85.3  Isc=6.09  Vm=72.9  Im=5.69  beta_Voc_pc=-0.229  alpha_Isc_pc=0.030706  beta_Voc=-0.19534  alpha_Isc=0.00187  IL=6.0978  I0=7.1698e-13  nI=0.87223  Rsh=419.7781  Rs=0.53711  RobustModel=off  RobustCellTemperature=313.3991  BAL=on  Tc=1e-6  Tfilter=5e-5
  RC_out : spsParallelRLCBranchLib/Parallel RLC Branch  LConnTagsString=a  RConnTagsString=__new0  BranchType=C  Resistance=30  Inductance=1e-3  SetiL0=off  InitialCurrent=0  Capacitance=239e-6  Setx0=off  InitialVoltage=700  Measurements=None
  Two-Level Converter : spsTwoLevelConverterLib/Two-Level Converter  ModelType=Average model (No rectifier mode)  Ron=1e-3  Rs=1e6  Cs=inf  Vforward=[0,0]  Ron_Diode=1e-3  Rs_Diode=1e6  Cs_Diode=inf  Vf_Diode=1e-3  Rs_CurrentSource=inf  Ron_ACsource=1e-3
  Voltage Measurement : spsVoltageMeasurementLib/Voltage Measurement  PhasorSimulation=off  OutputType=Complex  PSBequivalent=0
  A : PMIOPort  Side=Left
  B : PMIOPort  Port=2  Side=Left
  C : PMIOPort  Port=3  Side=Left
  tag scope: Vdc_meas_3=global, i_pv_3=global, v_pv_3=global
  wires:
  Bus Selector1/1 -> [v_pv_3]  "<V_PV>"
  Constant4/1 -> PV Array1/2
  Bus Selector1/2 -> [i_pv_3]  "<I_PV>"
  PV Array1/1 -> Bus Selector1/1
  [irr] -> PV Array1/1
  MPPT3/1(D) -> Boost Converter/1
  Inverter ON/OFF Logic/1(g_out) -> Two-Level Converter/1
  "  "/1 -> Inverter ON/OFF Logic/2(g_in)
  Voltage Measurement/1 -> Inverter ON/OFF Logic/1(V_DC), [Vdc_meas_3]
  connections:
  A/RConn1 -- Two-Level Converter/LConn1
  Two-Level Converter/RConn2 -- RC_out/RConn1 -- Voltage Measurement/LConn2 -- Boost Converter/RConn2 -- C_in/RConn1 -- PV Array1/RConn2
  C_in/LConn1 -- L_boost/LConn1 -- PV Array1/RConn1
  RC_out/LConn1 -- Two-Level Converter/RConn1 -- Boost Converter/RConn1 -- Voltage Measurement/LConn1
  C/RConn1 -- Two-Level Converter/LConn3
  B/RConn1 -- Two-Level Converter/LConn2
  L_boost/RConn1 -- Boost Converter/LConn1

== system Integration_1_1/VSC Control ==
  note: VSC Main Controller
  V : Inport  PortDimensions=3
  I : Inport  Port=2  PortDimensions=3
  Vdc : Inport  Port=3  PortDimensions=1
  Current Regulator : Subsystem
  Inverter ON/OFF Logic : Subsystem  Commented=through
  Iq_ref : Constant  Value=0
  Mux : Mux  Inputs=2
  PLL & Measurements : Subsystem
  PWM Generator (2-Level) : spsPWMGenerator2LevelLib/PWM Generator (2-Level)  Commented=through  ModulatorType=Three-phase bridge (6 pulses)  ModulatorMode=Unsynchronized  Fc=27*50*8  Pc=90  nF=27  MinMax="[ -1  1 ]"  SamplingTechnique=Natural  ModulatingSignals=off  m=0.8  Freq=60  Phase=0  Ts=Ts_Control  ShowCarrierOutport=off
  Product : Product
  Ramp : simulink/Sources/Ramp  slope=1/0.02  start=0  InitialOutput=0
  Saturation : Saturate  UpperLimit=1  LowerLimit=0
  Uabc_ref Generation max (m) = 1 : Subsystem
  Unit Delay : UnitDelay  SampleTime=Ts_Control  HasFrameUpgradeWarning=on
  VDC Regulator : Subsystem
  Vdc_ref1 : Constant  Value=Vdc_ref
  Uref : Outport  VectorParamsAs1DForOutWhenUnconnected=off
  wires:
  Vdc_ref1/1 -> VDC Regulator/2(Vdc_ref)
  Uabc_ref Generation max (m) = 1/1(Uabc_ref) -> Unit Delay/1
  Unit Delay/1 -> PWM Generator (2-Level)/1
  I/1 -> PLL & Measurements/2(Iabc_prim)
  V/1 -> PLL & Measurements/1(Vabc_prim)
  Vdc/1 -> VDC Regulator/1(Vdc_meas)
  PLL & Measurements/2(VdVq_prim) -> Current Regulator/1(VdVq_meas)
  PLL & Measurements/3(IdIq_prim) -> Current Regulator/2(IdIq_meas)
  Mux/1 -> Current Regulator/3(IdIq_ref)
  Iq_ref/1 -> Mux/2
  PLL & Measurements/1(wt) -> Uabc_ref Generation max (m) = 1/1(wt)
  VDC Regulator/1(Id_ref) -> Mux/1
  PWM Generator (2-Level)/1 -> Product/1
  Current Regulator/1(VdVq_conv) -> Uabc_ref Generation max (m) = 1/2(VdVq_conv)
  Product/1 -> Inverter ON/OFF Logic/1(V_DC)
  Ramp/1 -> Saturation/1
  Saturation/1 -> Product/2
  Inverter ON/OFF Logic/1(BL) -> Uref/1

== system Integration_1_1/VSC Control1 ==
  note: VSC Main Controller
  V : Inport  PortDimensions=3
  I : Inport  Port=2  PortDimensions=3
  Vdc : Inport  Port=3  PortDimensions=1
  Current Regulator : Subsystem
  Inverter ON/OFF Logic : Subsystem  Commented=through
  Iq_ref : Constant  Value=0
  Mux : Mux  Inputs=2
  PLL & Measurements : Subsystem
  PWM Generator (2-Level) : spsPWMGenerator2LevelLib/PWM Generator (2-Level)  Commented=through  ModulatorType=Three-phase bridge (6 pulses)  ModulatorMode=Unsynchronized  Fc=27*50*8  Pc=90  nF=27  MinMax="[ -1  1 ]"  SamplingTechnique=Natural  ModulatingSignals=off  m=0.8  Freq=60  Phase=0  Ts=Ts_Control  ShowCarrierOutport=off
  Product : Product
  Ramp : simulink/Sources/Ramp  slope=1/0.02  start=0  InitialOutput=0
  Saturation : Saturate  UpperLimit=1  LowerLimit=0
  Uabc_ref Generation max (m) = 1 : Subsystem
  Unit Delay : UnitDelay  SampleTime=Ts_Control  HasFrameUpgradeWarning=on
  VDC Regulator : Subsystem
  Vdc_ref1 : Constant  Value=Vdc_ref
  Uref : Outport  VectorParamsAs1DForOutWhenUnconnected=off
  wires:
  Vdc_ref1/1 -> VDC Regulator/2(Vdc_ref)
  Uabc_ref Generation max (m) = 1/1(Uabc_ref) -> Unit Delay/1
  Unit Delay/1 -> PWM Generator (2-Level)/1
  I/1 -> PLL & Measurements/2(Iabc_prim)
  V/1 -> PLL & Measurements/1(Vabc_prim)
  Vdc/1 -> VDC Regulator/1(Vdc_meas)
  PLL & Measurements/2(VdVq_prim) -> Current Regulator/1(VdVq_meas)
  PLL & Measurements/3(IdIq_prim) -> Current Regulator/2(IdIq_meas)
  Mux/1 -> Current Regulator/3(IdIq_ref)
  Iq_ref/1 -> Mux/2
  PLL & Measurements/1(wt) -> Uabc_ref Generation max (m) = 1/1(wt)
  VDC Regulator/1(Id_ref) -> Mux/1
  PWM Generator (2-Level)/1 -> Product/1
  Current Regulator/1(VdVq_conv) -> Uabc_ref Generation max (m) = 1/2(VdVq_conv)
  Product/1 -> Inverter ON/OFF Logic/1(V_DC)
  Ramp/1 -> Saturation/1
  Saturation/1 -> Product/2
  Inverter ON/OFF Logic/1(BL) -> Uref/1

== system Integration_1_1/VSC Control2 ==
  note: VSC Main Controller
  V : Inport  PortDimensions=3
  I : Inport  Port=2  PortDimensions=3
  Vdc : Inport  Port=3  PortDimensions=1
  Current Regulator : Subsystem
  Inverter ON/OFF Logic : Subsystem  Commented=through
  Iq_ref : Constant  Value=0
  Mux : Mux  Inputs=2
  PLL & Measurements : Subsystem
  PWM Generator (2-Level) : spsPWMGenerator2LevelLib/PWM Generator (2-Level)  Commented=through  ModulatorType=Three-phase bridge (6 pulses)  ModulatorMode=Unsynchronized  Fc=27*50*8  Pc=90  nF=27  MinMax="[ -1  1 ]"  SamplingTechnique=Natural  ModulatingSignals=off  m=0.8  Freq=60  Phase=0  Ts=Ts_Control  ShowCarrierOutport=off
  Product : Product
  Ramp : simulink/Sources/Ramp  slope=1/0.02  start=0  InitialOutput=0
  Saturation : Saturate  UpperLimit=1  LowerLimit=0
  Uabc_ref Generation max (m) = 1 : Subsystem
  Unit Delay : UnitDelay  SampleTime=Ts_Control  HasFrameUpgradeWarning=on
  VDC Regulator : Subsystem
  Vdc_ref1 : Constant  Value=Vdc_ref
  Uref : Outport  VectorParamsAs1DForOutWhenUnconnected=off
  wires:
  Inverter ON/OFF Logic/1(BL) -> Uref/1
  Saturation/1 -> Product/2
  Ramp/1 -> Saturation/1
  Product/1 -> Inverter ON/OFF Logic/1(V_DC)
  Current Regulator/1(VdVq_conv) -> Uabc_ref Generation max (m) = 1/2(VdVq_conv)
  PWM Generator (2-Level)/1 -> Product/1
  VDC Regulator/1(Id_ref) -> Mux/1
  PLL & Measurements/1(wt) -> Uabc_ref Generation max (m) = 1/1(wt)
  Iq_ref/1 -> Mux/2
  Mux/1 -> Current Regulator/3(IdIq_ref)
  PLL & Measurements/3(IdIq_prim) -> Current Regulator/2(IdIq_meas)
  PLL & Measurements/2(VdVq_prim) -> Current Regulator/1(VdVq_meas)
  Vdc/1 -> VDC Regulator/1(Vdc_meas)
  V/1 -> PLL & Measurements/1(Vabc_prim)
  I/1 -> PLL & Measurements/2(Iabc_prim)
  Unit Delay/1 -> PWM Generator (2-Level)/1
  Uabc_ref Generation max (m) = 1/1(Uabc_ref) -> Unit Delay/1
  Vdc_ref1/1 -> VDC Regulator/2(Vdc_ref)

== system Integration_1_1/VSC Control3 ==
  note: VSC Main Controller
  V : Inport  PortDimensions=3
  I : Inport  Port=2  PortDimensions=3
  Vdc : Inport  Port=3  PortDimensions=1
  Current Regulator : Subsystem
  Inverter ON/OFF Logic : Subsystem  Commented=through
  Iq_ref : Constant  Value=0
  Mux : Mux  Inputs=2
  PLL & Measurements : Subsystem
  PWM Generator (2-Level) : spsPWMGenerator2LevelLib/PWM Generator (2-Level)  Commented=through  ModulatorType=Three-phase bridge (6 pulses)  ModulatorMode=Unsynchronized  Fc=27*50*8  Pc=90  nF=27  MinMax="[ -1  1 ]"  SamplingTechnique=Natural  ModulatingSignals=off  m=0.8  Freq=60  Phase=0  Ts=Ts_Control  ShowCarrierOutport=off
  Product : Product
  Ramp : simulink/Sources/Ramp  slope=1/0.02  start=0  InitialOutput=0
  Saturation : Saturate  UpperLimit=1  LowerLimit=0
  Uabc_ref Generation max (m) = 1 : Subsystem
  Unit Delay : UnitDelay  SampleTime=Ts_Control  HasFrameUpgradeWarning=on
  VDC Regulator : Subsystem
  Vdc_ref1 : Constant  Value=Vdc_ref
  Uref : Outport  VectorParamsAs1DForOutWhenUnconnected=off
  wires:
  Inverter ON/OFF Logic/1(BL) -> Uref/1
  Saturation/1 -> Product/2
  Ramp/1 -> Saturation/1
  Product/1 -> Inverter ON/OFF Logic/1(V_DC)
  Current Regulator/1(VdVq_conv) -> Uabc_ref Generation max (m) = 1/2(VdVq_conv)
  PWM Generator (2-Level)/1 -> Product/1
  VDC Regulator/1(Id_ref) -> Mux/1
  PLL & Measurements/1(wt) -> Uabc_ref Generation max (m) = 1/1(wt)
  Iq_ref/1 -> Mux/2
  Mux/1 -> Current Regulator/3(IdIq_ref)
  PLL & Measurements/3(IdIq_prim) -> Current Regulator/2(IdIq_meas)
  PLL & Measurements/2(VdVq_prim) -> Current Regulator/1(VdVq_meas)
  Vdc/1 -> VDC Regulator/1(Vdc_meas)
  V/1 -> PLL & Measurements/1(Vabc_prim)
  I/1 -> PLL & Measurements/2(Iabc_prim)
  Unit Delay/1 -> PWM Generator (2-Level)/1
  Uabc_ref Generation max (m) = 1/1(Uabc_ref) -> Unit Delay/1
  Vdc_ref1/1 -> VDC Regulator/2(Vdc_ref)

== system Integration_1_1/VSC Control4 ==
  note: VSC Main Controller
  V : Inport  PortDimensions=3
  I : Inport  Port=2  PortDimensions=3
  Vdc : Inport  Port=3  PortDimensions=1
  Current Regulator : Subsystem
  Inverter ON/OFF Logic : Subsystem  Commented=through
  Iq_ref : Constant  Value=0
  Mux : Mux  Inputs=2
  PLL & Measurements : Subsystem
  PWM Generator (2-Level) : spsPWMGenerator2LevelLib/PWM Generator (2-Level)  Commented=through  ModulatorType=Three-phase bridge (6 pulses)  ModulatorMode=Unsynchronized  Fc=27*50*8  Pc=90  nF=27  MinMax="[ -1  1 ]"  SamplingTechnique=Natural  ModulatingSignals=off  m=0.8  Freq=60  Phase=0  Ts=Ts_Control  ShowCarrierOutport=off
  Product : Product
  Ramp : simulink/Sources/Ramp  slope=1/0.02  start=0  InitialOutput=0
  Saturation : Saturate  UpperLimit=1  LowerLimit=0
  Uabc_ref Generation max (m) = 1 : Subsystem
  Unit Delay : UnitDelay  SampleTime=Ts_Control  HasFrameUpgradeWarning=on
  VDC Regulator : Subsystem
  Vdc_ref1 : Constant  Value=Vdc_ref
  Uref : Outport  VectorParamsAs1DForOutWhenUnconnected=off
  wires:
  Vdc_ref1/1 -> VDC Regulator/2(Vdc_ref)
  Uabc_ref Generation max (m) = 1/1(Uabc_ref) -> Unit Delay/1
  Unit Delay/1 -> PWM Generator (2-Level)/1
  I/1 -> PLL & Measurements/2(Iabc_prim)
  V/1 -> PLL & Measurements/1(Vabc_prim)
  Vdc/1 -> VDC Regulator/1(Vdc_meas)
  PLL & Measurements/2(VdVq_prim) -> Current Regulator/1(VdVq_meas)
  PLL & Measurements/3(IdIq_prim) -> Current Regulator/2(IdIq_meas)
  Mux/1 -> Current Regulator/3(IdIq_ref)
  Iq_ref/1 -> Mux/2
  PLL & Measurements/1(wt) -> Uabc_ref Generation max (m) = 1/1(wt)
  VDC Regulator/1(Id_ref) -> Mux/1
  PWM Generator (2-Level)/1 -> Product/1
  Current Regulator/1(VdVq_conv) -> Uabc_ref Generation max (m) = 1/2(VdVq_conv)
  Product/1 -> Inverter ON/OFF Logic/1(V_DC)
  Ramp/1 -> Saturation/1
  Saturation/1 -> Product/2
  Inverter ON/OFF Logic/1(BL) -> Uref/1

== system Integration_1_1/VSC Control5 ==
  note: VSC Main Controller
  V : Inport  PortDimensions=3
  I : Inport  Port=2  PortDimensions=3
  Vdc : Inport  Port=3  PortDimensions=1
  Current Regulator : Subsystem
  Inverter ON/OFF Logic : Subsystem  Commented=through
  Iq_ref : Constant  Value=0
  Mux : Mux  Inputs=2
  PLL & Measurements : Subsystem
  PWM Generator (2-Level) : spsPWMGenerator2LevelLib/PWM Generator (2-Level)  Commented=through  ModulatorType=Three-phase bridge (6 pulses)  ModulatorMode=Unsynchronized  Fc=27*50*8  Pc=90  nF=27  MinMax="[ -1  1 ]"  SamplingTechnique=Natural  ModulatingSignals=off  m=0.8  Freq=60  Phase=0  Ts=Ts_Control  ShowCarrierOutport=off
  Product : Product
  Ramp : simulink/Sources/Ramp  slope=1/0.02  start=0  InitialOutput=0
  Saturation : Saturate  UpperLimit=1  LowerLimit=0
  Uabc_ref Generation max (m) = 1 : Subsystem
  Unit Delay : UnitDelay  SampleTime=Ts_Control  HasFrameUpgradeWarning=on
  VDC Regulator : Subsystem
  Vdc_ref1 : Constant  Value=Vdc_ref
  Uref : Outport  VectorParamsAs1DForOutWhenUnconnected=off
  wires:
  Inverter ON/OFF Logic/1(BL) -> Uref/1
  Saturation/1 -> Product/2
  Ramp/1 -> Saturation/1
  Product/1 -> Inverter ON/OFF Logic/1(V_DC)
  Current Regulator/1(VdVq_conv) -> Uabc_ref Generation max (m) = 1/2(VdVq_conv)
  PWM Generator (2-Level)/1 -> Product/1
  VDC Regulator/1(Id_ref) -> Mux/1
  PLL & Measurements/1(wt) -> Uabc_ref Generation max (m) = 1/1(wt)
  Iq_ref/1 -> Mux/2
  Mux/1 -> Current Regulator/3(IdIq_ref)
  PLL & Measurements/3(IdIq_prim) -> Current Regulator/2(IdIq_meas)
  PLL & Measurements/2(VdVq_prim) -> Current Regulator/1(VdVq_meas)
  Vdc/1 -> VDC Regulator/1(Vdc_meas)
  V/1 -> PLL & Measurements/1(Vabc_prim)
  I/1 -> PLL & Measurements/2(Iabc_prim)
  Unit Delay/1 -> PWM Generator (2-Level)/1
  Uabc_ref Generation max (m) = 1/1(Uabc_ref) -> Unit Delay/1
  Vdc_ref1/1 -> VDC Regulator/2(Vdc_ref)

== system Integration_1_1/Scopes/SoC ==
  I : Inport
  Compare To Constant : simulink/Logic and Bit Operations/Compare To Constant  relop===  const=36  OutDataTypeStr=boolean
  Compare To Constant1 : simulink/Logic and Bit Operations/Compare To Constant  relop=>=  const=54  OutDataTypeStr=boolean
  Compare To Constant2 : simulink/Logic and Bit Operations/Compare To Constant  relop=>=  const=100  OutDataTypeStr=boolean
  Constant : Constant  Value=0
  Constant1 : Constant
  D Flip-Flop : simulink_extras/Flip Flops/D Flip-Flop
  Gain1 : Gain  Gain=-21600
  Gain2 : Gain  Gain=1/360000
  Gain3 : Gain  Gain=100
  Integrator : Integrator  ExternalReset=rising
  Saturation : Saturate  UpperLimit=1  LowerLimit=0
  Switch : Switch  Criteria=u2 > Threshold  SaturateOnIntegerOverflow=off  InputSameDT=off
  Switch1 : Switch  Criteria=u2 > Threshold  SaturateOnIntegerOverflow=off  InputSameDT=off
  SoC : Outport
  wires:
  I/1 -> Gain1/1
  Gain1/1 -> Integrator/1
  Gain2/1 -> Saturation/1
  Integrator/1 -> Gain2/1
  Gain3/1 -> Compare To Constant2/1, SoC/1
  [Batt_V] -> Compare To Constant1/1, Compare To Constant/1
  Compare To Constant/1 -> Switch/2
  Constant/1 -> Switch/1
  Saturation/1 -> Switch/3
  Switch1/1 -> Gain3/1
  Switch/1 -> Switch1/3
  Compare To Constant1/1 -> Switch1/2
  Constant1/1 -> Switch1/1
  D Flip-Flop/1 -> Integrator/2
  Compare To Constant2/1 -> D Flip-Flop/1

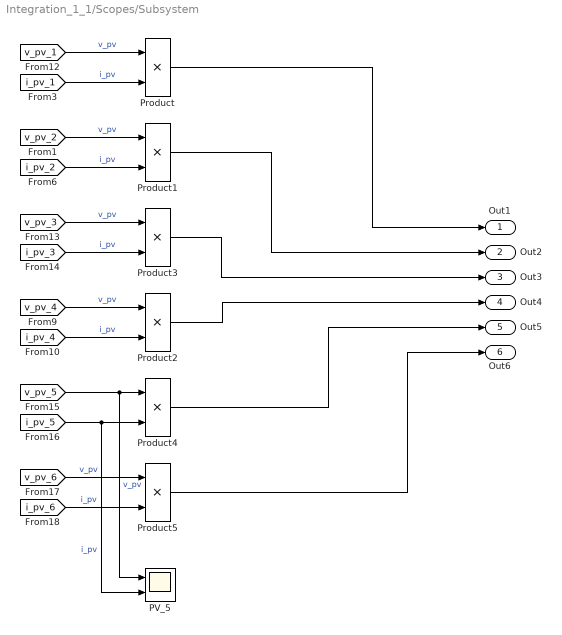
== system Integration_1_1/Scopes/Subsystem ==
  PV_5 : Scope  NumInputPorts=2
  Product{,1..5} (6 alike) : Product
  Out1 : Outport
  Out2 : Outport  Port=2
  Out3 : Outport  Port=3
  Out4 : Outport  Port=4
  Out5 : Outport  Port=5
  Out6 : Outport  Port=6
  wires:
  [i_pv_1] -> Product/2  "i_pv"
  [v_pv_2] -> Product1/1  "v_pv"
  [v_pv_1] -> Product/1  "v_pv"
  [i_pv_3] -> Product3/2  "i_pv"
  [v_pv_3] -> Product3/1  "v_pv"
  [i_pv_6] -> Product5/2  "i_pv"
  [v_pv_6] -> Product5/1  "v_pv"
  [i_pv_2] -> Product1/2  "i_pv"
  [v_pv_4] -> Product2/1  "v_pv"
  [i_pv_4] -> Product2/2  "i_pv"
  [v_pv_5] -> PV_5/1, Product4/1  "v_pv"
  [i_pv_5] -> PV_5/2, Product4/2  "i_pv"
  Product/1 -> Out1/1
  Product1/1 -> Out2/1
  Product2/1 -> Out4/1
  Product3/1 -> Out3/1
  Product4/1 -> Out5/1
  Product5/1 -> Out6/1

== system Integration_1_1/Subsystem/Inverter ON//OFF Logic ==
  V_DC : Inport
  g_in : Inport  Port=2
  Compare To Constant : simulink/Logic and Bit Operations/Compare To Constant  relop=>  const=600  OutDataTypeStr=boolean
  Data Type Conversion : DataTypeConversion  OutDataTypeStr=double  SaturateOnIntegerOverflow=off  RndMeth=Floor
  Product : Product
  Unit Delay : UnitDelay  SampleTime=-1  HasFrameUpgradeWarning=on
  g_out : Outport
  wires:
  Data Type Conversion/1 -> Product/1
  V_DC/1 -> Compare To Constant/1
  Compare To Constant/1 -> Data Type Conversion/1
  Product/1 -> Unit Delay/1
  g_in/1 -> Product/2
  Unit Delay/1 -> g_out/1
